simulink model "myo_sfun_two_myo_imu"  (R2013a)
settings: Solver=ode1  StartTime=0.0  StopTime=inf  FixedStep=0.02  RelTol=1e-3
libraries: myo_lib x3, rtwinlib x1
settings Model: Creator=Mark Tomaszewski  LastModifiedBy=marktoma
settings OptimizationCC: InlineParams=on
settings GRTTargetCC: ExtMode=on

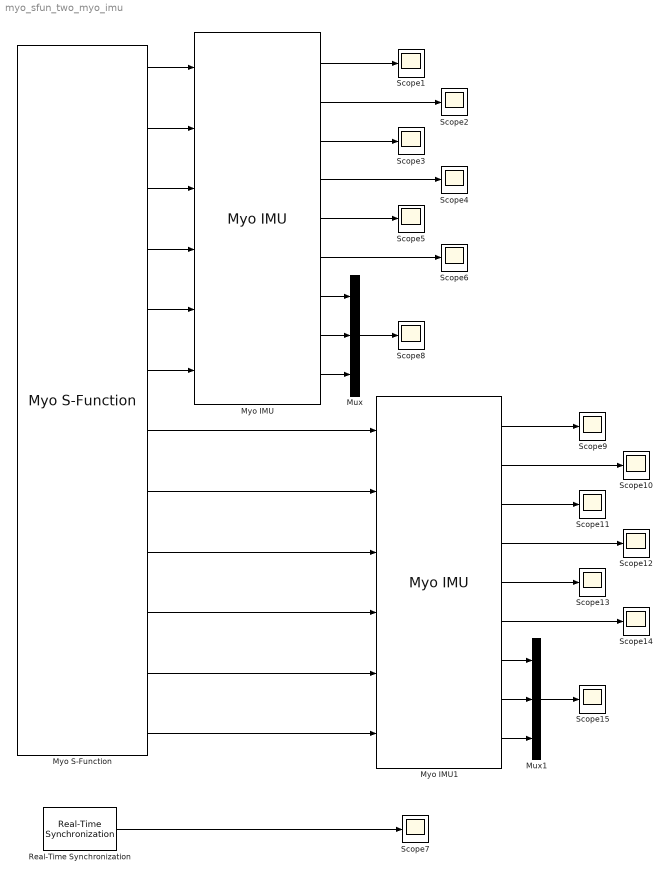
== system myo_sfun_two_myo_imu ==
  Mux : Mux  Inputs=3
  Mux1 : Mux  Inputs=3
  Myo IMU : myo_lib/Myo IMU
  Myo IMU1 : myo_lib/Myo IMU
  Myo S-Function : myo_lib/Myo S-Function  emgEnabled=0  countMyos=2
  Real-Time Synchronization : rtwinlib/Real-Time Synchronization  SampleTime=0.04  MaxMissedTicks=50  ShowMissedTicks=on  YieldWhenWaiting=on
  Scope{1..15} (15 alike) : Scope
      Scope1 settings: TimeRange=10  YMin=-150  YMax=150
      Scope10 settings: TimeRange=10  YMin=-150  YMax=150  SaveName=ScopeData8
      Scope11 settings: TimeRange=10  YMin=-150  YMax=150  SaveName=ScopeData9
      Scope12 settings: TimeRange=10  YMin=-150  YMax=150  SaveName=ScopeData10
      Scope13 settings: TimeRange=10  YMin=-150  YMax=150  SaveName=ScopeData11
      Scope14 settings: TimeRange=10  YMin=-150  YMax=150  SaveName=ScopeData12
      Scope15 settings: TimeRange=10  YMin=-150  YMax=150  SaveName=ScopeData13
      Scope2 settings: TimeRange=10  YMin=-150  YMax=150
      Scope3 settings: TimeRange=10  YMin=-150  YMax=150  SaveName=ScopeData2
      Scope4 settings: TimeRange=10  YMin=-150  YMax=150  SaveName=ScopeData3
      Scope5 settings: TimeRange=10  YMin=-150  YMax=150  SaveName=ScopeData4
      Scope6 settings: TimeRange=10  YMin=-150  YMax=150  SaveName=ScopeData5
      Scope7 settings: TimeRange=10  YMin=-150  YMax=150  SaveName=ScopeData7
      Scope8 settings: TimeRange=10  YMin=-150  YMax=150  SaveName=ScopeData6
      Scope9 settings: TimeRange=10  YMin=-150  YMax=150  SaveName=ScopeData14
  wires:
  Real-Time Synchronization/1 -> Scope7/1
  Myo S-Function/3 -> Myo IMU/3
  Myo S-Function/2 -> Myo IMU/2
  Myo S-Function/4 -> Myo IMU/4
  Myo S-Function/1 -> Myo IMU/1
  Myo S-Function/5 -> Myo IMU/5
  Myo S-Function/6 -> Myo IMU/6
  Myo S-Function/8 -> Myo IMU1/2
  Myo S-Function/10 -> Myo IMU1/4
  Myo S-Function/9 -> Myo IMU1/3
  Myo S-Function/12 -> Myo IMU1/6
  Myo S-Function/11 -> Myo IMU1/5
  Myo S-Function/7 -> Myo IMU1/1
  Myo IMU/1 -> Scope1/1
  Myo IMU/2 -> Scope2/1
  Myo IMU/3 -> Scope3/1
  Myo IMU/4 -> Scope4/1
  Myo IMU/5 -> Scope5/1
  Myo IMU/6 -> Scope6/1
  Myo IMU/8 -> Mux/2
  Myo IMU/9 -> Mux/3
  Myo IMU/7 -> Mux/1
  Mux/1 -> Scope8/1
  Myo IMU1/1 -> Scope9/1
  Myo IMU1/2 -> Scope10/1
  Myo IMU1/3 -> Scope11/1
  Myo IMU1/4 -> Scope12/1
  Myo IMU1/5 -> Scope13/1
  Myo IMU1/6 -> Scope14/1
  Myo IMU1/8 -> Mux1/2
  Myo IMU1/7 -> Mux1/1
  Mux1/1 -> Scope15/1
  Myo IMU1/9 -> Mux1/3
